simulink model "cx06_MA"  (Simulink 7.5)
settings: Solver=FixedStepDiscrete  StartTime=0.0  StopTime=10.0  RelTol=1e-3
undefined symbols (not defined in the file or in its folder): DiscIntNeverNeededParam, ECU555, int, motohawk_build_version, motohawk_trunc_name, motohawk_vardec_path
libraries: MotoHawk_lib x811, simulink x43, simulink_need_slupdate x1
(part 2 of 10)

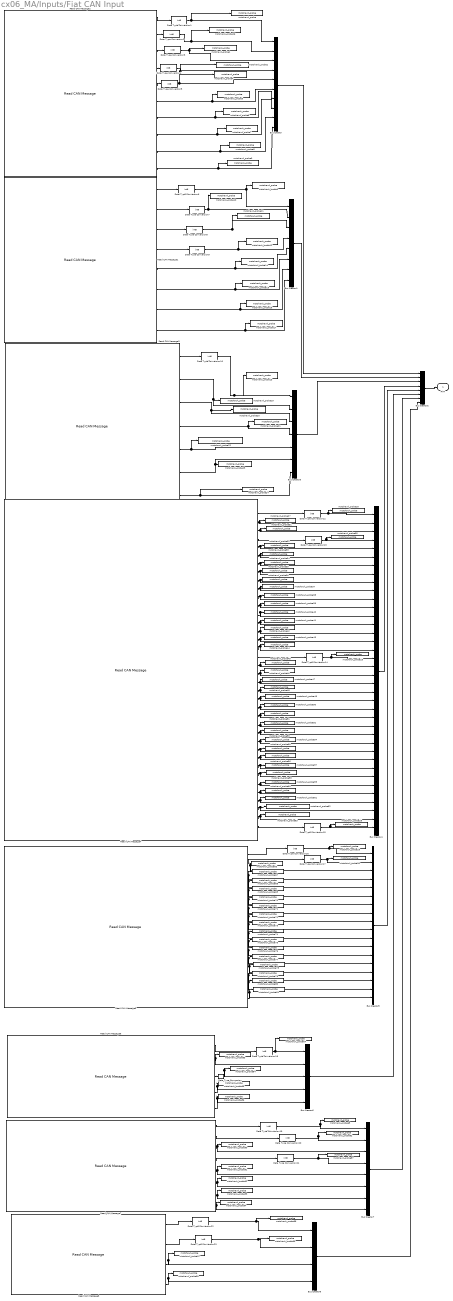
== system cx06_MA/Inputs/Fiat CAN Input ==
  Bus Creator : BusCreator  Inputs=10
  Bus Creator1 : BusCreator  Inputs=8
  Bus Creator2 : BusCreator  Inputs=8
  Bus Creator3 : BusCreator  Inputs=7
  Bus Creator4 : BusCreator  Inputs=38
  Bus Creator5 : BusCreator  Inputs=18
  Bus Creator6 : BusCreator  Inputs=5
  Bus Creator7 : BusCreator  Inputs=8
  Bus Creator8 : BusCreator
  Data Type Conversion : DataTypeConversion  OutDataTypeMode=uint8  OutDataType=sfix(16)  OutScaling=2^0  OutDataTypeStr=uint8
  Data Type Conversion{1..10,12..23} (22 alike) : DataTypeConversion  OutDataTypeMode=int8  OutDataType=sfix(16)  OutScaling=2^0  OutDataTypeStr=int8
  Read CAN Message1 : MotoHawk_lib/CAN Blocks/Read CAN Message  nam=['CAN_' num2str(1)]  bus=-2  msg=CANRx_FIAT_120  queue=2  slot=''  valid=off  stale=off  labelwires=on
  Read CAN Message2 : MotoHawk_lib/CAN Blocks/Read CAN Message  nam=['CAN_' num2str(1)]  bus=-2  msg=CANRx_FIAT_110  queue=2  slot=''  valid=off  stale=off  labelwires=on
  Read CAN Message3 : MotoHawk_lib/CAN Blocks/Read CAN Message  nam=['CAN_' num2str(1)]  bus=-2  msg=CANRx_FIAT_1A0  queue=2  slot=''  valid=off  stale=off  labelwires=on
  Read CAN Message4 : MotoHawk_lib/CAN Blocks/Read CAN Message  nam=['CAN_' num2str(1)]  bus=-2  msg=CANRx_FIAT_300  queue=2  slot=''  valid=off  stale=off  labelwires=on
  Read CAN Message5 : MotoHawk_lib/CAN Blocks/Read CAN Message  nam=['CAN_' num2str(1)]  bus=-2  msg=CANRx_FIAT_301  queue=2  slot=''  valid=off  stale=off  labelwires=on
  Read CAN Message6 : MotoHawk_lib/CAN Blocks/Read CAN Message  nam=['CAN_' num2str(1)]  bus=-2  msg=CANRx_FIAT_348  queue=2  slot=''  valid=off  stale=off  labelwires=on
  Read CAN Message7 : MotoHawk_lib/CAN Blocks/Read CAN Message  nam=['CAN_' num2str(1)]  bus=-2  msg=CANRx_FIAT_410  queue=2  slot=''  valid=off  stale=off  labelwires=on
  Read CAN Message8 : MotoHawk_lib/CAN Blocks/Read CAN Message  nam=['CAN_' num2str(1)]  bus=-2  msg=CANRx_FIAT_510  queue=2  slot=''  valid=off  stale=off  labelwires=on
  motohawk_probe{,1..3,10..13,18,25..26,28..30,64..65,82,87..89,95} (21 alike) : MotoHawk_lib/Calibration & Probing Blocks/motohawk_probe  nam='Probe'  show_more=on  name_source=Use Input Wire Name  read_level=1  view_as=Enumeration  enum_struct={'Valid', 'Invalid'}  vector_style=Wide Row  use_help_units=off  help=''  units=''  use_header_enum=off  row_header_enum={}  col_header_enum={}  use_precision=off  precision=''  gain=1  offset=0  exp=1  use_mototune_group=on  mototune_group=[motohawk_vardec_path(gcb), ' | Validities']
  motohawk_probe{5..8,14..17,19..20,24} (11 alike) : MotoHawk_lib/Calibration & Probing Blocks/motohawk_probe  nam='Probe'  show_more=off  name_source=Use Input Wire Name  read_level=1  view_as=Number  enum_struct={'Disabled', 'Enabled'}  vector_style=Wide Row  use_help_units=off  help=''  units=''  use_header_enum=off  row_header_enum={}  col_header_enum={}  use_precision=off  precision=''  gain=1  offset=0  exp=1  use_mototune_group=off  mototune_group=motohawk_vardec_path(gcb)
  motohawk_probe21 : MotoHawk_lib/Calibration & Probing Blocks/motohawk_probe  nam='Probe'  show_more=on  name_source=Use Input Wire Name  read_level=1  view_as=Number  enum_struct={'Status Unknown', 'Backup Mode Inactive', 'Backup Mode Active','Data Invalid'}  vector_style=Wide Row  use_help_units=off  help=''  units=''  use_header_enum=off  row_header_enum={}  col_header_enum={}  use_precision=off  precision=''  gain=1  offset=0  exp=1  use_mototune_group=off  mototune_group=motohawk_vardec_path(gcb)
  motohawk_probe22 : MotoHawk_lib/Calibration & Probing Blocks/motohawk_probe  nam='Probe'  show_more=on  name_source=Use Input Wire Name  read_level=1  view_as=Number  enum_struct={'Status Unknown', 'Normal Operation Without Failures','Reduced Power Mode Active','Power Management Mode Active','Safety Fuel Shut-Off Mode Active','Forced Idle Mode Active','Bowden Cable Mode Active','Engine Shut-Down Mode Active'}  vector_style=Wide Row  use_help_units=off  help=''  units=''  use_header_enum=off  row_header_enum={}  col_header_enum={}  use_precision=off  precision=''  gain=1  offset=0  exp=1  use_mototune_group=off  mototune_group=motohawk_vardec_path(gcb)
  motohawk_probe23 : MotoHawk_lib/Calibration & Probing Blocks/motohawk_probe  nam='Probe'  show_more=on  name_source=Use Input Wire Name  read_level=1  view_as=Number  enum_struct={'Status Unknown','Backup Mode Inactive','Backup Mode Active','Data Invalid'}  vector_style=Wide Row  use_help_units=off  help=''  units=''  use_header_enum=off  row_header_enum={}  col_header_enum={}  use_precision=off  precision=''  gain=1  offset=0  exp=1  use_mototune_group=off  mototune_group=motohawk_vardec_path(gcb)
  motohawk_probe{27,31..38,41..42,47..58,60..63,66..68,70..74,83,90..94,97..98} (43 alike) : MotoHawk_lib/Calibration & Probing Blocks/motohawk_probe  nam='Probe'  show_more=on  name_source=Use Input Wire Name  read_level=1  view_as=Number  enum_struct={'Valid','Invalid'}  vector_style=Wide Row  use_help_units=on  help=''  units=''  use_header_enum=off  row_header_enum={}  col_header_enum={}  use_precision=off  precision=''  gain=1  offset=0  exp=1  use_mototune_group=off  mototune_group=motohawk_vardec_path(gcb)
  motohawk_probe39 : MotoHawk_lib/Calibration & Probing Blocks/motohawk_probe  nam='Probe'  show_more=on  name_source=Use Input Wire Name  read_level=1  view_as=Number  enum_struct={'Not Running','Running and Idling','Running and Not Idling'}  vector_style=Wide Row  use_help_units=on  help=''  units=''  use_header_enum=off  row_header_enum={}  col_header_enum={}  use_precision=off  precision=''  gain=1  offset=0  exp=1  use_mototune_group=off  mototune_group=motohawk_vardec_path(gcb)
  motohawk_probe4 : MotoHawk_lib/Calibration & Probing Blocks/motohawk_probe  nam='Probe'  show_more=on  name_source=Use Input Wire Name  read_level=1  view_as=Enumeration  enum_struct={'Invalid','Valid'}  vector_style=Wide Row  use_help_units=off  help=''  units=''  use_header_enum=off  row_header_enum={}  col_header_enum={}  use_precision=off  precision=''  gain=1  offset=0  exp=1  use_mototune_group=on  mototune_group=[motohawk_vardec_path(gcb), ' | Validities']
  motohawk_probe40 : MotoHawk_lib/Calibration & Probing Blocks/motohawk_probe  nam='Probe'  show_more=on  name_source=Use Input Wire Name  read_level=1  view_as=Number  enum_struct={'Inactive','Active'}  vector_style=Wide Row  use_help_units=on  help=''  units=''  use_header_enum=off  row_header_enum={}  col_header_enum={}  use_precision=off  precision=''  gain=1  offset=0  exp=1  use_mototune_group=off  mototune_group=motohawk_vardec_path(gcb)
  motohawk_probe43 : MotoHawk_lib/Calibration & Probing Blocks/motohawk_probe  nam='Probe'  show_more=on  name_source=Use Input Wire Name  read_level=1  view_as=Number  enum_struct={'No Indication','Continuous Indication','Flashing Indication'}  vector_style=Wide Row  use_help_units=on  help=''  units=''  use_header_enum=off  row_header_enum={}  col_header_enum={}  use_precision=off  precision=''  gain=1  offset=0  exp=1  use_mototune_group=off  mototune_group=motohawk_vardec_path(gcb)
  motohawk_probe44 : MotoHawk_lib/Calibration & Probing Blocks/motohawk_probe  nam='Probe'  show_more=on  name_source=Use Input Wire Name  read_level=1  view_as=Number  enum_struct={'Cruise Not Active','Cruise Control In Command','Driver Overriding Cruise Command','Higher Priority Function Overriding'}  vector_style=Wide Row  use_help_units=on  help=''  units=''  use_header_enum=off  row_header_enum={}  col_header_enum={}  use_precision=off  precision=''  gain=1  offset=0  exp=1  use_mototune_group=off  mototune_group=motohawk_vardec_path(gcb)
  motohawk_probe45 : MotoHawk_lib/Calibration & Probing Blocks/motohawk_probe  nam='Probe'  show_more=on  name_source=Use Input Wire Name  read_level=1  view_as=Number  enum_struct={'Brake Not Applied','Brake Applied'}  vector_style=Wide Row  use_help_units=on  help=''  units=''  use_header_enum=off  row_header_enum={}  col_header_enum={}  use_precision=off  precision=''  gain=1  offset=0  exp=1  use_mototune_group=off  mototune_group=motohawk_vardec_path(gcb)
  motohawk_probe46 : MotoHawk_lib/Calibration & Probing Blocks/motohawk_probe  nam='Probe'  show_more=on  name_source=Use Input Wire Name  read_level=1  view_as=Number  enum_struct={'Brake Not Applied','Brake Applied'}  vector_style=Wide Row  use_help_units=on  help=''  units=''  use_header_enum=off  row_header_enum={}  col_header_enum={}  use_precision=off  precision=''  gain=1  offset=0  exp=1  use_mototune_group=off  mototune_group=motohawk_vardec_path(gcb)
  motohawk_probe59 : MotoHawk_lib/Calibration & Probing Blocks/motohawk_probe  nam='Probe'  show_more=on  name_source=Use Input Wire Name  read_level=1  view_as=Number  enum_struct={'Limited Slip Control Permitted','Limited Slip Control Inhibited'}  vector_style=Wide Row  use_help_units=on  help=''  units=''  use_header_enum=off  row_header_enum={}  col_header_enum={}  use_precision=off  precision=''  gain=1  offset=0  exp=1  use_mototune_group=off  mototune_group=motohawk_vardec_path(gcb)
  motohawk_probe69 : MotoHawk_lib/Calibration & Probing Blocks/motohawk_probe  nam='Probe'  show_more=on  name_source=Use Input Wire Name  read_level=1  view_as=Number  enum_struct={'None','Shift Up','Shift Down','Neutral'}  vector_style=Wide Row  use_help_units=on  help=''  units=''  use_header_enum=off  row_header_enum={}  col_header_enum={}  use_precision=off  precision=''  gain=1  offset=0  exp=1  use_mototune_group=off  mototune_group=motohawk_vardec_path(gcb)
  motohawk_probe75 : MotoHawk_lib/Calibration & Probing Blocks/motohawk_probe  nam='Probe'  show_more=on  name_source=Use Input Wire Name  read_level=1  view_as=Number  enum_struct={'No Request','Inhibit Gear Shift'}  vector_style=Wide Row  use_help_units=on  help=''  units=''  use_header_enum=off  row_header_enum={}  col_header_enum={}  use_precision=off  precision=''  gain=1  offset=0  exp=1  use_mototune_group=off  mototune_group=motohawk_vardec_path(gcb)
  motohawk_probe76 : MotoHawk_lib/Calibration & Probing Blocks/motohawk_probe  nam='Probe'  show_more=on  name_source=Use Input Wire Name  read_level=1  view_as=Number  enum_struct={'No Request','Request Jerk Shift Pattern'}  vector_style=Wide Row  use_help_units=on  help=''  units=''  use_header_enum=off  row_header_enum={}  col_header_enum={}  use_precision=off  precision=''  gain=1  offset=0  exp=1  use_mototune_group=off  mototune_group=motohawk_vardec_path(gcb)
  motohawk_probe77 : MotoHawk_lib/Calibration & Probing Blocks/motohawk_probe  nam='Probe'  show_more=on  name_source=Use Input Wire Name  read_level=1  view_as=Number  enum_struct={'No Request','Inhibit Neutral Control'}  vector_style=Wide Row  use_help_units=on  help=''  units=''  use_header_enum=off  row_header_enum={}  col_header_enum={}  use_precision=off  precision=''  gain=1  offset=0  exp=1  use_mototune_group=off  mototune_group=motohawk_vardec_path(gcb)
  motohawk_probe78 : MotoHawk_lib/Calibration & Probing Blocks/motohawk_probe  nam='Probe'  show_more=on  name_source=Use Input Wire Name  read_level=1  view_as=Number  enum_struct={'No Request','Request REP Shift Pattern'}  vector_style=Wide Row  use_help_units=on  help=''  units=''  use_header_enum=off  row_header_enum={}  col_header_enum={}  use_precision=off  precision=''  gain=1  offset=0  exp=1  use_mototune_group=off  mototune_group=motohawk_vardec_path(gcb)
  motohawk_probe79 : MotoHawk_lib/Calibration & Probing Blocks/motohawk_probe  nam='Probe'  show_more=on  name_source=Use Input Wire Name  read_level=1  view_as=Number  enum_struct={'Map A','Map B','Map C','ECM Selected Progression'}  vector_style=Wide Row  use_help_units=on  help=''  units=''  use_header_enum=off  row_header_enum={}  col_header_enum={}  use_precision=off  precision=''  gain=1  offset=0  exp=1  use_mototune_group=off  mototune_group=motohawk_vardec_path(gcb)
  motohawk_probe80 : MotoHawk_lib/Calibration & Probing Blocks/motohawk_probe  nam='Probe'  show_more=on  name_source=Use Input Wire Name  read_level=1  view_as=Number  enum_struct={'Map A','Map B','Map C','ECM Selected Progression'}  vector_style=Wide Row  use_help_units=on  help=''  units=''  use_header_enum=off  row_header_enum={}  col_header_enum={}  use_precision=off  precision=''  gain=1  offset=0  exp=1  use_mototune_group=off  mototune_group=motohawk_vardec_path(gcb)
  motohawk_probe81 : MotoHawk_lib/Calibration & Probing Blocks/motohawk_probe  nam='Probe'  show_more=on  name_source=Use Input Wire Name  read_level=1  view_as=Number  enum_struct={'Map A','Map B','Map C','ECM Selected Progression'}  vector_style=Wide Row  use_help_units=on  help=''  units=''  use_header_enum=off  row_header_enum={}  col_header_enum={}  use_precision=off  precision=''  gain=1  offset=0  exp=1  use_mototune_group=off  mototune_group=motohawk_vardec_path(gcb)
  motohawk_probe84 : MotoHawk_lib/Calibration & Probing Blocks/motohawk_probe  nam='Probe'  show_more=on  name_source=Use Input Wire Name  read_level=1  view_as=Enumeration  enum_struct={'No Action','Engage','Minimum Stroke','Security Shutdown'}  vector_style=Wide Row  use_help_units=on  help=''  units=''  use_header_enum=off  row_header_enum={}  col_header_enum={}  use_precision=off  precision=''  gain=1  offset=0  exp=1  use_mototune_group=off  mototune_group=motohawk_vardec_path(gcb)
  motohawk_probe85 : MotoHawk_lib/Calibration & Probing Blocks/motohawk_probe  nam='Probe'  show_more=on  name_source=Use Input Wire Name  read_level=1  view_as=Number  enum_struct={'No Action','Engage','Minimum Stroke','Security Shutdown'}  vector_style=Wide Row  use_help_units=on  help=''  units=''  use_header_enum=off  row_header_enum={}  col_header_enum={}  use_precision=off  precision=''  gain=1  offset=0  exp=1  use_mototune_group=off  mototune_group=motohawk_vardec_path(gcb)
  motohawk_probe86 : MotoHawk_lib/Calibration & Probing Blocks/motohawk_probe  nam='Probe'  show_more=on  name_source=Use Input Wire Name  read_level=1  view_as=Number  enum_struct={'No Action','Engage','Minimum Stroke','Security Shutdown'}  vector_style=Wide Row  use_help_units=on  help=''  units=''  use_header_enum=off  row_header_enum={}  col_header_enum={}  use_precision=off  precision=''  gain=1  offset=0  exp=1  use_mototune_group=off  mototune_group=motohawk_vardec_path(gcb)
  motohawk_probe9 : MotoHawk_lib/Calibration & Probing Blocks/motohawk_probe  nam='Probe'  show_more=on  name_source=Use Input Wire Name  read_level=1  view_as=Number  enum_struct={'Disabled', 'Enabled'}  vector_style=Wide Row  use_help_units=off  help=''  units=''  use_header_enum=off  row_header_enum={}  col_header_enum={}  use_precision=off  precision=''  gain=1  offset=0  exp=1  use_mototune_group=off  mototune_group=motohawk_vardec_path(gcb)
  FIAT : Outport  OutDataType=sfix(16)  OutScaling=2^0
  wires:
  Read CAN Message2/1 -> Data Type Conversion1/1  "Eng_Spd_V"
  Read CAN Message2/2 -> Data Type Conversion2/1  "Acel_Effect_Pos_V"
  Read CAN Message2/3 -> Data Type Conversion3/1  "Acel_Grad_V"
  Read CAN Message2/4 -> Data Type Conversion4/1  "Throt_Pos_V"
  Bus Creator/1 -> Bus Creator2/1  "Engine Speed and Pedal Pos"
  Bus Creator2/1 -> FIAT/1
  Read CAN Message2/5 -> Data Type Conversion5/1  "Acel_Actual_Pos_V"
  Read CAN Message2/7 -> Bus Creator/7, motohawk_probe6/1  "Acel_Effect_Pos"
  Read CAN Message2/8 -> Bus Creator/8, motohawk_probe7/1  "Acel_Grad"
  Read CAN Message2/9 -> Bus Creator/9, motohawk_probe8/1  "Throt_Pos"
  Read CAN Message2/10 -> Bus Creator/10, motohawk_probe9/1  "Acel_Actual_Pos"
  Read CAN Message1/1 -> Data Type Conversion6/1  "Eng_Torq_Actual_V"
  Read CAN Message1/2 -> Data Type Conversion7/1  "Eng_Torq_Driver_Reqest_V"
  Read CAN Message1/3 -> Data Type Conversion8/1  "Eng_Max_Drag_Torq_V"
  Read CAN Message1/4 -> Data Type Conversion9/1  "Eng_Torq_Max_V"
  Read CAN Message1/5 -> Bus Creator1/5, motohawk_probe14/1  "Eng_Torq_Actual"
  Read CAN Message1/6 -> Bus Creator1/6, motohawk_probe15/1  "Eng_Torq_Request"
  Read CAN Message1/7 -> Bus Creator1/7, motohawk_probe16/1  "Eng_Max_Drag_Torq"
  Read CAN Message1/8 -> Bus Creator1/8, motohawk_probe17/1  "Eng_Torq_Max"
  Bus Creator1/1 -> Bus Creator2/2  "Engine Torque"
  Read CAN Message2/6 -> Bus Creator/6, motohawk_probe5/1  "Eng_Spd"
  Read CAN Message3/1 -> Data Type Conversion10/1  "Eng_Idle_Spd_V"
  Read CAN Message3/2 -> Bus Creator3/2, motohawk_probe19/1  "Eng_Idle_Spd"
  Read CAN Message3/3 -> Bus Creator3/3, motohawk_probe20/1  "Base_Target_Eng_Idle_Spd"
  Read CAN Message3/4 -> Bus Creator3/4, motohawk_probe21/1  "Eng_Airflow_Backup_Mode"
  Read CAN Message3/5 -> Bus Creator3/5, motohawk_probe22/1  "Eng_Throt_Control_Operat"
  Read CAN Message3/6 -> Bus Creator3/6, motohawk_probe23/1  "Eng_Crankshaft_Backup_Mode"
  Read CAN Message3/7 -> Bus Creator3/7, motohawk_probe24/1  "Eng_Allowed_Clutch_Adapt"
  Bus Creator3/1 -> Bus Creator2/3  "Engine Idle Speed Info"
  Read CAN Message4/1 -> Data Type Conversion12/1  "Brake_Ped_Switch_Active_V"
  Read CAN Message4/2 -> Bus Creator4/2, motohawk_probe27/1  "Part_Filter_Clean_Alg_Active"
  Read CAN Message4/3 -> Bus Creator4/3, motohawk_probe31/1  "Fuel_Inj_Roll_Cnt_Reset_Occured"
  Read CAN Message4/5 -> Bus Creator4/5, motohawk_probe32/1  "Eng_Limp_Home_Mode"
  Read CAN Message4/6 -> Bus Creator4/6, motohawk_probe33/1  "Eng_Torq_Reduction_Failed"
  Read CAN Message4/7 -> Bus Creator4/7, motohawk_probe34/1  "Eng_Fail_Code_Retrieval_Required"
  Read CAN Message4/8 -> Bus Creator4/8, motohawk_probe35/1  "Generator_Failed"
  Read CAN Message4/9 -> Bus Creator4/9, motohawk_probe36/1  "Brake_Ped_Switch"
  Read CAN Message4/10 -> Bus Creator4/10, motohawk_probe37/1  "Cruise_Control_Clutch_Switch"
  Read CAN Message4/11 -> Bus Creator4/11, motohawk_probe38/1  "Cruise_Control_Active"
  Read CAN Message4/12 -> Bus Creator4/12, motohawk_probe39/1  "Eng_Running_Stat"
  Read CAN Message4/13 -> Bus Creator4/13, motohawk_probe40/1  "Warm_Up_Shift_Pattern_Req"
  Read CAN Message4/14 -> Bus Creator4/14, motohawk_probe41/1  "Rough_Road"
  Read CAN Message4/15 -> Bus Creator4/15, motohawk_probe42/1  "Eng_Warm_Up_Cycle_Achieved"
  Read CAN Message4/16 -> Bus Creator4/16, motohawk_probe43/1  "Service_Eng_Non_Emission"
  Read CAN Message4/17 -> Bus Creator4/17, motohawk_probe44/1  "Cruise_Control_Throt_Cmd_Stat"
  Read CAN Message4/19 -> Bus Creator4/19, motohawk_probe45/1  "PwrTrn_Brk_Ped_Sec_In"
  Read CAN Message4/20 -> Bus Creator4/20, motohawk_probe46/1  "PrwTrn_Brk_Ped_In"
  Read CAN Message4/21 -> Bus Creator4/21, motohawk_probe47/1  "Eng_Oil_Lvl_Low"
  Read CAN Message4/22 -> Bus Creator4/22, motohawk_probe48/1  "Eng_Oil_Pres_Low"
  Read CAN Message4/23 -> Bus Creator4/23, motohawk_probe49/1  "Accel_Kick_Down"
  Read CAN Message4/24 -> motohawk_probe50/1, Bus Creator4/24  "Glow_Plug"
  Read CAN Message4/25 -> Bus Creator4/25, motohawk_probe51/1  "PrwTrn_Crank"
  Read CAN Message4/26 -> Bus Creator4/26, motohawk_probe52/1  "Eng_Trans_Emission_DTC_Stored"
  Read CAN Message4/27 -> Bus Creator4/27, motohawk_probe53/1  "Eng_Torq_Tract_Control_Req_Failed"
  Read CAN Message4/28 -> Bus Creator4/28, motohawk_probe54/1  "Eng_Torq_Trans_Req_Failed"
  Read CAN Message4/29 -> Bus Creator4/29, motohawk_probe55/1  "Fuel_Inj_Roll_Cnt"
  Read CAN Message4/30 -> Bus Creator4/30, motohawk_probe56/1  "Fuel_Lvl_Sensor_Unprocessed"
  Read CAN Message4/31 -> Bus Creator4/31, motohawk_probe57/1  "Eng_Emissions_Malfunction"
  Read CAN Message4/32 -> Bus Creator4/32, motohawk_probe58/1  "Cruise_Control_Enabled"
  Read CAN Message4/33 -> Bus Creator4/33, motohawk_probe59/1  "Eng_Coast_Limit_Slip"
  Read CAN Message4/34 -> Bus Creator4/34, motohawk_probe60/1  "Eng_Oil_Change_Now"
  Read CAN Message4/35 -> Bus Creator4/35, motohawk_probe61/1  "Eng_Oil_Change_Soon"
  Read CAN Message4/36 -> Bus Creator4/36, motohawk_probe62/1  "Eng_Coast_Fuel_Cut_Off_Active"
  Read CAN Message4/37 -> Bus Creator4/37, motohawk_probe63/1  "Eng_Torq_Cruise_Control_Req_Failed"
  Read CAN Message4/38 -> Data Type Conversion15/1  "PwrTrn_Brk_Ped_In_V"
  Read CAN Message4/4 -> Data Type Conversion13/1  "Fuel_Lvl_Sensor_Unprocessed_Value_V"
  Read CAN Message5/2 -> Data Type Conversion17/1  "Baro_Pres_Abs_V"
  Read CAN Message5/3 -> motohawk_probe66/1, Bus Creator5/3  "PwrTrn_Hi_Elect_Load_Req"
  Read CAN Message5/4 -> motohawk_probe67/1, Bus Creator5/4  "Aply_Brk_Pedal_Ind"
  Read CAN Message5/5 -> motohawk_probe68/1, Bus Creator5/5  "Check_Fuel_Cap"
  Read CAN Message5/6 -> motohawk_probe69/1, Bus Creator5/6  "Eng_Recommend_Shft"
  Read CAN Message5/7 -> motohawk_probe70/1, Bus Creator5/7  "Eng_H20_In_Fuel"
  Read CAN Message5/8 -> motohawk_probe71/1, Bus Creator5/8  "Eng_Boost_Pres"
  Read CAN Message5/9 -> motohawk_probe72/1, Bus Creator5/9  "Eng_Oil_Remaining_Life"
  Read CAN Message5/10 -> motohawk_probe73/1, Bus Creator5/10  "Eng_Prod_Option_Ident"
  Read CAN Message5/11 -> motohawk_probe74/1, Bus Creator5/11  "Eng_Fan_Spd"
  Read CAN Message5/12 -> motohawk_probe75/1, Bus Creator5/12  "Eng_Gear_Shift_Inh_Req"
  Read CAN Message5/13 -> motohawk_probe76/1, Bus Creator5/13  "Eng_Jerk_Shift_Pattern_Req"
  Read CAN Message5/14 -> motohawk_probe77/1, Bus Creator5/14  "Eng_Ntral_Control_Inh_Req"
  Read CAN Message5/15 -> motohawk_probe78/1, Bus Creator5/15  "Reduce_Prf_Shft_Ptrn_Req"
  Read CAN Message5/16 -> motohawk_probe79/1, Bus Creator5/16  "Throt_Progression"
  Read CAN Message5/17 -> motohawk_probe80/1, Bus Creator5/17  "PwrTrn_Part_Filter Warning"
  Read CAN Message5/18 -> motohawk_probe81/1, Bus Creator5/18  "Baro_Pres_Abs"
  Read CAN Message6/1 -> Data Type Conversion18/1  "AC_Ref_Hi_Side_Pres_V"
  Read CAN Message6/2 -> motohawk_probe83/1, Bus Creator6/2  "AC_Comp_Clutch_Engaged"
  Read CAN Message6/3 -> Data Type Conversion/1  "AC_Comp_Stroke_Req"
  Read CAN Message6/4 -> motohawk_probe85/1, Bus Creator6/4  "AC_Off_Ind"
  Read CAN Message6/5 -> motohawk_probe86/1, Bus Creator6/5  "AC_Ref_Hi_Side_Pres"
  Read CAN Message7/1 -> Data Type Conversion19/1  "Veh_Spd_V"
  Read CAN Message7/2 -> Data Type Conversion20/1  "Dist_Roll_Cnt_Lft_V"
  Read CAN Message7/4 -> Data Type Conversion21/1  "Dist_Roll_Cnt_Rht_V"
  Read CAN Message7/3 -> motohawk_probe90/1, Bus Creator7/3  "Dist_Roll_Cnt_Lft_Reset"
  Read CAN Message7/5 -> motohawk_probe91/1, Bus Creator7/5  "Dist_Roll_Cnt_Rht_Reset"
  Read CAN Message7/6 -> motohawk_probe92/1, Bus Creator7/6  "Veh_Spd"
  Read CAN Message7/7 -> motohawk_probe93/1, Bus Creator7/7  "Dist_Roll_Cnt_Lft"
  Read CAN Message7/8 -> motohawk_probe94/1, Bus Creator7/8  "Dist_Roll_Cnt_Rht"
  Read CAN Message8/3 -> motohawk_probe97/1, Bus Creator8/3  "Eng_Coolant_Temp"
  Read CAN Message8/4 -> motohawk_probe98/1, Bus Creator8/4  "Eng_Intake_Air_Temp"
  Bus Creator4/1 -> Bus Creator2/4  "Engine  General Status"
  Bus Creator5/1 -> Bus Creator2/5  "Engine General Status 2"
  Bus Creator6/1 -> Bus Creator2/6  "Engine AC Status"
  Bus Creator7/1 -> Bus Creator2/7  "Vehicle Speed and Odometer"
  Bus Creator8/1 -> Bus Creator2/8  "Engine Temp"
  Data Type Conversion/1 -> motohawk_probe84/1, Bus Creator6/3  "AC_Comp_Stroke_Req"
  Data Type Conversion1/1 -> Bus Creator/1, motohawk_probe/1  "Eng_Spd_V"
  Data Type Conversion2/1 -> Bus Creator/2, motohawk_probe26/1  "Acel_Effect_Pos_V"
  Data Type Conversion3/1 -> Bus Creator/3, motohawk_probe1/1  "Acel_Grad_V"
  Data Type Conversion4/1 -> Bus Creator/4, motohawk_probe2/1  "Throt_Pos_V"
  Data Type Conversion5/1 -> Bus Creator/5, motohawk_probe4/1  "Acel_Actual_Pos_V"
  Data Type Conversion6/1 -> Bus Creator1/1, motohawk_probe3/1  "Eng_Torq_Actual_V"
  Data Type Conversion7/1 -> Bus Creator1/2, motohawk_probe10/1  "Eng_Torq_Driver_Reqest_V"
  Data Type Conversion8/1 -> Bus Creator1/3, motohawk_probe11/1  "Eng_Max_Drag_Torq_V"
  Data Type Conversion9/1 -> Bus Creator1/4, motohawk_probe12/1  "Eng_Torq_Max_V"
  Data Type Conversion10/1 -> Bus Creator3/1, motohawk_probe13/1  "Eng_Idle_Spd_V"
  Data Type Conversion12/1 -> Bus Creator4/1, motohawk_probe18/1  "Brake_Ped_Switch_Active_V"
  Data Type Conversion13/1 -> Bus Creator4/4, motohawk_probe95/1  "Fuel_Lvl_Sensor_Unprocessed_Value_V"
  Read CAN Message4/18 -> Data Type Conversion14/1  "PwrTrn_Brk_Ped_Sec_In_V"
  Data Type Conversion14/1 -> Bus Creator4/18, motohawk_probe25/1  "PwrTrn_Brk_Ped_Sec_In_V"
  Data Type Conversion15/1 -> Bus Creator4/38, motohawk_probe28/1  "PwrTrn_Brk_Ped_In_V"
  Read CAN Message5/1 -> Data Type Conversion16/1  "Eng_Boost_Pres_V"
  Data Type Conversion16/1 -> Bus Creator5/1, motohawk_probe29/1  "Eng_Boost_Pres_V"
  Data Type Conversion17/1 -> Bus Creator5/2, motohawk_probe30/1  "Baro_Pres_Abs_V"
  Data Type Conversion18/1 -> Bus Creator6/1, motohawk_probe64/1  "AC_Ref_Hi_Side_Pres_V"
  Data Type Conversion19/1 -> Bus Creator7/1, motohawk_probe65/1  "Veh_Spd_V"
  Data Type Conversion20/1 -> Bus Creator7/2, motohawk_probe82/1  "Dist_Roll_Cnt_Lft_V"
  Data Type Conversion21/1 -> Bus Creator7/4, motohawk_probe87/1  "Dist_Roll_Cnt_Rht_V"
  Read CAN Message8/1 -> Data Type Conversion22/1  "Eng_Coolant_Temp_V"
  Data Type Conversion22/1 -> Bus Creator8/1, motohawk_probe88/1  "Eng_Coolant_Temp_V"
  Read CAN Message8/2 -> Data Type Conversion23/1  "Eng_Intake_Air_Temp_V"
  Data Type Conversion23/1 -> Bus Creator8/2, motohawk_probe89/1  "Eng_Intake_Air_Temp_V"

== system cx06_MA/Inputs/GMLAN Inputs ==
  Bus Creator : BusCreator  Inputs=10
  Compare To Constant1 : simulink/Logic and Bit Operations/Compare To Constant  SystemSampleTime=-1  relop=>  const=10  LogicOutDataTypeMode=boolean  ZeroCross=off
  Compare To Constant2 : simulink/Logic and Bit Operations/Compare To Constant  SystemSampleTime=-1  relop=>  const=20  LogicOutDataTypeMode=boolean  ZeroCross=off
  Read CAN Message : MotoHawk_lib/CAN Blocks/Read CAN Message  nam=['CAN_' num2str(2)]  bus=-2  msg=CANRx_GMLAN_280  queue=1  slot=''  valid=off  stale=on  labelwires=on
  Read CAN Message1 : MotoHawk_lib/CAN Blocks/Read CAN Message  nam=['CAN_' num2str(2)]  bus=-2  msg=CANRx_GMLAN_380  queue=1  slot=''  valid=off  stale=on  labelwires=on
  Valid_Chk : Subsystem
  Valid_Chk1 : Subsystem
  Valid_Chk2 : Subsystem
  Valid_Chk3 : Subsystem
  motohawk_fault_def1 : MotoHawk_lib/Fault Management Blocks/motohawk_fault_def  nam='GMLAN380'  mode=Enabled - Persistent  id=[]  x=10  y=11  input_suspected=on  indeterminate=off  increment_xy=on  downsample_count=1  ovr_cals=on  ovr_actions=on  show_actions=on  action1_name=''  action1_cond=(None)  action2_name=''  action2_cond=(None)  action3_name=''  action3_cond=(None)  action4_name=''  action4_cond=(None)
  motohawk_fault_def2 : MotoHawk_lib/Fault Management Blocks/motohawk_fault_def  nam='GMLAN280'  mode=Enabled - Persistent  id=[]  x=10  y=11  input_suspected=on  indeterminate=off  increment_xy=on  downsample_count=1  ovr_cals=on  ovr_actions=on  show_actions=on  action1_name=''  action1_cond=(None)  action2_name=''  action2_cond=(None)  action3_name=''  action3_cond=(None)  action4_name=''  action4_cond=(None)
  motohawk_probe{,1..12} (13 alike) : MotoHawk_lib/Calibration & Probing Blocks/motohawk_probe  nam='Probe'  show_more=on  name_source=Use Input Wire Name  read_level=1  view_as=Number  enum_struct={'Disabled', 'Enabled'}  vector_style=Wide Row  use_help_units=off  help=''  units=''  use_header_enum=off  row_header_enum={}  col_header_enum={}  use_precision=off  precision=''  gain=1  offset=0  exp=1  use_mototune_group=off  mototune_group=motohawk_vardec_path(gcb)
  GMLAN : Outport  OutDataType=sfix(16)  OutScaling=2^0
  wires:
  Valid_Chk/1(Out1) -> Bus Creator/2  "FL_Whl_Spd"
  Valid_Chk1/1(Out1) -> Bus Creator/3  "FR_Whl_Spd"
  Valid_Chk2/1(Out1) -> Bus Creator/4  "RL_Whl_Spd"
  Valid_Chk3/1(Out1) -> Bus Creator/5  "RR_Whl_Spd"
  Compare To Constant2/1 -> motohawk_fault_def2/1  "AgeCount"
  Read CAN Message/1 -> Compare To Constant2/1, Bus Creator/1  "AgeCount"
  Read CAN Message/2 -> motohawk_probe/1, Valid_Chk/1(In)  "FL_Wheel_Vel"
  Read CAN Message/3 -> motohawk_probe1/1, Valid_Chk/2(Valid)  "FL_Wheel_Valid"
  Read CAN Message/4 -> motohawk_probe2/1, Valid_Chk1/1(In)  "FR_Wheel_Vel"
  Read CAN Message/5 -> motohawk_probe3/1, Valid_Chk1/2(Valid)  "FR_Wheel_Valid"
  Read CAN Message/6 -> motohawk_probe4/1, Valid_Chk2/1(In)  "RL_Wheel_Vel"
  Read CAN Message/7 -> motohawk_probe5/1, Valid_Chk2/2(Valid)  "RL_Wheel_Valid"
  Read CAN Message/8 -> motohawk_probe6/1, Valid_Chk3/1(In)  "RR_Wheel_Vel"
  Read CAN Message/9 -> motohawk_probe7/1, Valid_Chk3/2(Valid)  "RR_Wheel_Valid"
  Compare To Constant1/1 -> motohawk_fault_def1/1  "AgeCount"
  Read CAN Message1/1 -> Compare To Constant1/1  "AgeCount"
  Read CAN Message1/2 -> motohawk_probe8/1, Bus Creator/6  "AC_Clutch_Req"
  Read CAN Message1/3 -> motohawk_probe9/1, Bus Creator/7  "System_Power_Mode"
  Read CAN Message1/4 -> motohawk_probe10/1, Bus Creator/8  "RunCrank_Status"
  Read CAN Message1/5 -> motohawk_probe11/1, Bus Creator/9  "Acc_Status"
  Bus Creator/1 -> GMLAN/1  "GMLAN"
  Read CAN Message1/6 -> Bus Creator/10, motohawk_probe12/1  "Park_Brake"

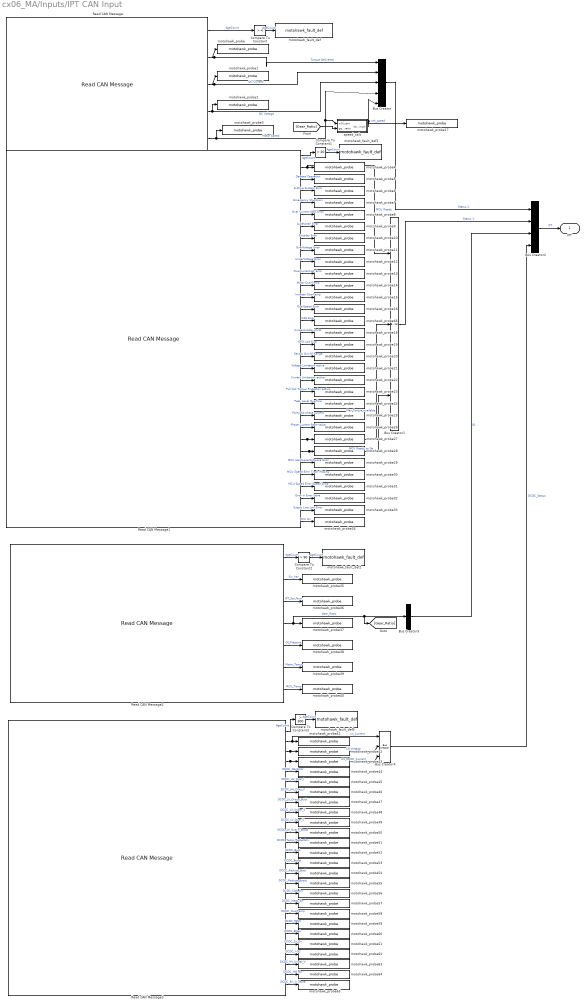
== system cx06_MA/Inputs/IPT CAN Input ==
  Bus Creator : BusCreator  Inputs=5
  Bus Creator1 : BusCreator  Inputs=3
  Bus Creator2 : BusCreator
  Bus Creator3 : BusCreator  Inputs=1
  Bus Creator4 : BusCreator  Inputs=3
  Compare To Constant : simulink/Logic and Bit Operations/Compare To Constant  SystemSampleTime=-1  relop=>  const=4  LogicOutDataTypeMode=boolean  ZeroCross=off
  Compare To Constant1 : simulink/Logic and Bit Operations/Compare To Constant  SystemSampleTime=-1  relop=>  const=20  LogicOutDataTypeMode=boolean  ZeroCross=off
  Compare To Constant2 : simulink/Logic and Bit Operations/Compare To Constant  SystemSampleTime=-1  relop=>  const=90  LogicOutDataTypeMode=boolean  ZeroCross=off
  Compare To Constant3 : simulink/Logic and Bit Operations/Compare To Constant  SystemSampleTime=-1  relop=>  const=300  LogicOutDataTypeMode=boolean  ZeroCross=off
  Read CAN Message : MotoHawk_lib/CAN Blocks/Read CAN Message  nam=['CAN_' num2str(1)]  bus=-2  msg=CANRx_IPT_258  queue=2  slot=''  valid=off  stale=on  labelwires=on
  Read CAN Message1 : MotoHawk_lib/CAN Blocks/Read CAN Message  nam=['CAN_' num2str(1)]  bus=-2  msg=CANRx_IPT_278  queue=2  slot=''  valid=off  stale=on  labelwires=on
  Read CAN Message2 : MotoHawk_lib/CAN Blocks/Read CAN Message  nam=['CAN_' num2str(1)]  bus=-2  msg=CANRx_IPT_638  queue=1  slot=''  valid=off  stale=on  labelwires=on
  Read CAN Message3 : MotoHawk_lib/CAN Blocks/Read CAN Message  nam=['CAN_' num2str(1)]  bus=-2  msg=CANRx_IPT_620  queue=1  slot=''  valid=off  stale=on  labelwires=on
  motohawk_fault_def : MotoHawk_lib/Fault Management Blocks/motohawk_fault_def  nam='IPT258'  mode=Enabled - Persistent  id=[]  x=10  y=11  input_suspected=on  indeterminate=off  increment_xy=on  downsample_count=1  ovr_cals=on  ovr_actions=on  show_actions=on  action1_name=''  action1_cond=Active  action2_name='inhibitEV'  action2_cond=Active  action3_name=''  action3_cond=(None)  action4_name=''  action4_cond=(None)
  motohawk_fault_def1 : MotoHawk_lib/Fault Management Blocks/motohawk_fault_def  nam='IPT278'  mode=Enabled - Persistent  id=[]  x=10  y=11  input_suspected=on  indeterminate=off  increment_xy=on  downsample_count=1  ovr_cals=on  ovr_actions=on  show_actions=on  action1_name=''  action1_cond=Active  action2_name='inhibitEV'  action2_cond=Active  action3_name=''  action3_cond=(None)  action4_name=''  action4_cond=(None)
  motohawk_fault_def2 : MotoHawk_lib/Fault Management Blocks/motohawk_fault_def  nam='IPT638'  mode=Enabled - Persistent  id=[]  x=10  y=11  input_suspected=on  indeterminate=off  increment_xy=on  downsample_count=1  ovr_cals=on  ovr_actions=on  show_actions=on  action1_name='inhibitEV'  action1_cond=Active  action2_name=''  action2_cond=(None)  action3_name=''  action3_cond=(None)  action4_name=''  action4_cond=(None)
  motohawk_fault_def3 : MotoHawk_lib/Fault Management Blocks/motohawk_fault_def  nam='IPT620'  mode=Enabled - Persistent  id=[]  x=29  y=30  input_suspected=on  indeterminate=off  increment_xy=on  downsample_count=1  ovr_cals=on  ovr_actions=on  show_actions=on  action1_name=''  action1_cond=Active  action2_name=''  action2_cond=(None)  action3_name=''  action3_cond=(None)  action4_name=''  action4_cond=(None)
  motohawk_probe : MotoHawk_lib/Calibration & Probing Blocks/motohawk_probe  nam='Probe'  show_more=on  name_source=Use Input Wire Name  read_level=1  view_as=Number  enum_struct={'Disabled', 'Enabled'}  vector_style=Wide Row  use_help_units=off  help=''  units=''  use_header_enum=off  row_header_enum={}  col_header_enum={}  use_precision=off  precision=''  gain=1  offset=0  exp=1  use_mototune_group=off  mototune_group=motohawk_vardec_path(gcb)
  motohawk_probe1 : MotoHawk_lib/Calibration & Probing Blocks/motohawk_probe  nam='Probe'  show_more=on  name_source=Use Input Wire Name  read_level=1  view_as=Number  enum_struct={'Disabled', 'Enabled'}  vector_style=Wide Row  use_help_units=off  help=''  units=''  use_header_enum=off  row_header_enum={}  col_header_enum={}  use_precision=off  precision=''  gain=1  offset=0  exp=1  use_mototune_group=off  mototune_group=motohawk_vardec_path(gcb)
  motohawk_probe{3..16,18..66} (63 alike) : MotoHawk_lib/Calibration & Probing Blocks/motohawk_probe  nam='Probe'  show_more=off  name_source=Use Input Wire Name  read_level=1  view_as=Number  enum_struct={'Disabled', 'Enabled'}  vector_style=Wide Row  use_help_units=off  help=''  units=''  use_header_enum=off  row_header_enum={}  col_header_enum={}  use_precision=off  precision=''  gain=1  offset=0  exp=1  use_mototune_group=off  mototune_group=motohawk_vardec_path(gcb)
  motohawk_probe17 : MotoHawk_lib/Calibration & Probing Blocks/motohawk_probe  nam='vehicle_speed'  show_more=on  name_source=Use Parameter  read_level=1  view_as=Number  enum_struct={'Disabled', 'Enabled'}  vector_style=Wide Row  use_help_units=off  help=''  units=''  use_header_enum=off  row_header_enum={}  col_header_enum={}  use_precision=off  precision=''  gain=1  offset=0  exp=1  use_mototune_group=off  mototune_group=motohawk_vardec_path(gcb)
  motohawk_probe2 : MotoHawk_lib/Calibration & Probing Blocks/motohawk_probe  nam='Probe'  show_more=on  name_source=Use Input Wire Name  read_level=1  view_as=Number  enum_struct={'Disabled', 'Enabled'}  vector_style=Wide Row  use_help_units=off  help=''  units=''  use_header_enum=off  row_header_enum={}  col_header_enum={}  use_precision=off  precision=''  gain=1  offset=0  exp=1  use_mototune_group=off  mototune_group=motohawk_vardec_path(gcb)
  speed_calc : Subsystem
  IPT : Outport  OutDataType=sfix(16)  OutScaling=2^0
  wires:
  Bus Creator/1 -> Bus Creator2/1  "Status 2"
  Bus Creator1/1 -> Bus Creator2/2  "Status 1"
  Bus Creator2/1 -> IPT/1  "IPT"
  Bus Creator3/1 -> Bus Creator2/3  "ID"
  Bus Creator4/1 -> Bus Creator2/4  "DCDC_Status"
  Compare To Constant/1 -> motohawk_fault_def/1  "AgeCount"
  Read CAN Message/2 -> Bus Creator/1, motohawk_probe/1  "Torque Delivered"
  Read CAN Message/3 -> Bus Creator/2, motohawk_probe1/1  "DC Current"
  Read CAN Message/5 -> motohawk_probe3/1, Bus Creator/4, speed_calc/1(whl_rpm)  "Motor Speed"
  Read CAN Message/1 -> Compare To Constant/1  "AgeCount"
  Read CAN Message/4 -> Bus Creator/3, motohawk_probe2/1  "DC Voltage"
  Compare To Constant1/1 -> motohawk_fault_def1/1  "AgeCount"
  Read CAN Message1/1 -> Compare To Constant1/1  "AgeCount"
  Read CAN Message1/2 -> motohawk_probe4/1, Bus Creator1/1  "MCU Ready"
  Read CAN Message1/3 -> motohawk_probe5/1  "Derated Operation"
  Read CAN Message1/4 -> motohawk_probe6/1  "E-Drive System Error"
  Read CAN Message1/5 -> motohawk_probe7/1  "Emergency Shutdown"
  Read CAN Message1/6 -> motohawk_probe8/1  "Over Current IGBT Error"
  Read CAN Message1/7 -> motohawk_probe9/1  "Lube(Anal) Error"
  Read CAN Message1/8 -> motohawk_probe10/1  "Encoder Error"
  Read CAN Message1/9 -> motohawk_probe11/1  "OverVoltage Error"
  Read CAN Message1/10 -> motohawk_probe12/1  "UnderVoltage Error"
  Read CAN Message1/11 -> motohawk_probe13/1  "OverCurrent-AC Error"
  Read CAN Message1/12 -> motohawk_probe14/1  "Motor OverTemp"
  Read CAN Message1/13 -> motohawk_probe15/1  "Inverter OverTemp"
  Read CAN Message1/14 -> motohawk_probe16/1  "OverSpeed Error"
  Read CAN Message1/15 -> motohawk_probe66/1  "CAN Error"
  Read CAN Message1/16 -> motohawk_probe18/1  "Unreasonable Limits"
  Read CAN Message1/17 -> motohawk_probe19/1  "EPO Line Error"
  Read CAN Message1/18 -> motohawk_probe20/1  "Sensor Out Of Range"
  Read CAN Message1/19 -> motohawk_probe21/1  "Voltage Limitation active"
  Read CAN Message1/20 -> motohawk_probe22/1  "Current Limitiation active"
  Read CAN Message1/21 -> motohawk_probe23/1  "Pull Out Torque Protection active"
  Read CAN Message1/22 -> motohawk_probe24/1  "Peak Level Overflow"
  Read CAN Message1/23 -> motohawk_probe25/1  "Parity bit phase current"
  Read CAN Message1/24 -> motohawk_probe26/1  "Phase Current Peak-Value"
  Read CAN Message1/25 -> motohawk_probe27/1, Bus Creator1/2  "Max Torque available"
  Read CAN Message1/26 -> motohawk_probe28/1, Bus Creator1/3  "MCU Ready to Go"
  Read CAN Message1/27 -> motohawk_probe29/1  "MCU Hardware/Software Error"
  Read CAN Message1/28 -> motohawk_probe30/1  "MCU Speed Error Track Missing"
  Read CAN Message1/29 -> motohawk_probe31/1  "MCU Speed Error Speed Jump"
  Read CAN Message1/30 -> motohawk_probe32/1  "Error in Error Store"
  Read CAN Message1/31 -> motohawk_probe33/1  "Supply Line Low Error"
  Read CAN Message1/32 -> motohawk_probe34/1  "MCU On"
  Compare To Constant2/1 -> motohawk_fault_def2/1  "AgeCount"
  Read CAN Message2/1 -> Compare To Constant2/1  "AgeCount"
  Read CAN Message2/2 -> motohawk_probe35/1  "Sw_Ver"
  Read CAN Message2/3 -> motohawk_probe36/1  "IPT_Ser_Num"
  Read CAN Message2/4 -> motohawk_probe37/1, Bus Creator3/1, [Gear_Ratio]  "Gear_Ratio"
  Read CAN Message2/5 -> motohawk_probe38/1  "Oil_Pressure"
  Read CAN Message2/6 -> motohawk_probe39/1  "Motor_Temp"
  Read CAN Message2/7 -> motohawk_probe40/1  "MCU_Temp"
  Compare To Constant3/1 -> motohawk_fault_def3/1  "AgeCount"
  Read CAN Message3/1 -> Compare To Constant3/1  "AgeCount"
  Read CAN Message3/2 -> motohawk_probe41/1, Bus Creator4/1  "LV_Current"
  Read CAN Message3/3 -> motohawk_probe42/1, Bus Creator4/2  "LV_Voltage"
  Read CAN Message3/4 -> motohawk_probe43/1, Bus Creator4/3  "HV_DCDC_Current"
  Read CAN Message3/5 -> motohawk_probe44/1  "DCDC_GenError"
  Read CAN Message3/6 -> motohawk_probe45/1  "DCDC_HV_Over_I"
  Read CAN Message3/7 -> motohawk_probe46/1  "DCDC_HV_Over_V"
  Read CAN Message3/8 -> motohawk_probe47/1  "DCDC_LV_Over_I_Buck"
  Read CAN Message3/9 -> motohawk_probe48/1  "DCDC_LV_Under_V"
  Read CAN Message3/10 -> motohawk_probe49/1  "DCDC_LV_Over_V"
  Read CAN Message3/11 -> motohawk_probe50/1  "DCDC_LV_Over_I_Boost"
  Read CAN Message3/12 -> motohawk_probe51/1  "DCDC_Temp_Reduction"
  Read CAN Message3/13 -> motohawk_probe52/1  "DCDC_Buck"
  Read CAN Message3/14 -> motohawk_probe53/1  "DCDC_Boost"
  Read CAN Message3/15 -> motohawk_probe54/1  "DCDC_Reduce_Buck"
  Read CAN Message3/16 -> motohawk_probe55/1  "DCDC_Reduce_Boost"
  Read CAN Message3/17 -> motohawk_probe56/1  "DCDC_CAN_Err"
  Read CAN Message3/18 -> motohawk_probe57/1  "DCDC_Meas_Err"
  Read CAN Message3/19 -> motohawk_probe58/1  "DCDC_OverTemp"
  Read CAN Message3/20 -> motohawk_probe59/1  "DCDC_90I2t"
  Read CAN Message3/21 -> motohawk_probe60/1  "DCDC_Break"
  Read CAN Message3/22 -> motohawk_probe61/1  "DCDC_3x_En"
  Read CAN Message3/23 -> motohawk_probe62/1  "DCDC_>0C"
  Read CAN Message3/24 -> motohawk_probe63/1  "DCDC_HV_Under_V"
  Read CAN Message3/25 -> motohawk_probe64/1  "DCDC_HW_Err"
  Read CAN Message3/26 -> motohawk_probe65/1  "DCDC_Err_in_Store"
  speed_calc/1(Veh_mph) -> Bus Creator/5, motohawk_probe17/1  "veh_speed"
  [Gear_Ratio] -> speed_calc/2(gear_ratio)

== system cx06_MA/Inputs/JCI CAN Input ==
  Bus Creator3 : BusCreator
  Read CAN Message : MotoHawk_lib/CAN Blocks/Read CAN Message  nam=['CAN_' num2str(2)]  bus=-2  msg=CANRx_JCS_300  queue=1  slot=''  valid=off  stale=off  labelwires=on
  Read CAN Message1 : MotoHawk_lib/CAN Blocks/Read CAN Message  nam=['CAN_' num2str(2)]  bus=-2  msg=CANRx_JCS_310  queue=2  slot=''  valid=off  stale=off  labelwires=on
  SOC : Stateflow chart  TreatAsAtomicUnit=on
  Unit Delay : UnitDelay  SampleTime=-1
  motohawk_calibration : MotoHawk_lib/Calibration & Probing Blocks/motohawk_calibration  nam='cuurentPlusMinus'  val=3.25  storage=Calibration  show_more=on  name_source=Use Parameter  data_type=double  read_level=1  write_level=1  ovr_cals=on  view_as=Number  enum_struct={'Disabled', 'Enabled'}  vector_style=Wide Row  use_help_units=off  help=''  units=''  use_header_enum=off  row_header_enum={}  col_header_enum={}  use_min_max=off  min_val=-inf  max_val=inf  use_precision=off  precision=''  gain=1  offset=0  exp=1  use_mototune_group=off  mototune_group=motohawk_vardec_path(gcb)
  motohawk_calibration1 : MotoHawk_lib/Calibration & Probing Blocks/motohawk_calibration  nam='lowV'  val=195  storage=Calibration  show_more=on  name_source=Use Parameter  data_type=double  read_level=1  write_level=1  ovr_cals=on  view_as=Number  enum_struct={'Disabled', 'Enabled'}  vector_style=Wide Row  use_help_units=off  help=''  units=''  use_header_enum=off  row_header_enum={}  col_header_enum={}  use_min_max=off  min_val=-inf  max_val=inf  use_precision=off  precision=''  gain=1  offset=0  exp=1  use_mototune_group=off  mototune_group=motohawk_vardec_path(gcb)
  motohawk_calibration2 : MotoHawk_lib/Calibration & Probing Blocks/motohawk_calibration  nam='highV'  val=285  storage=Calibration  show_more=on  name_source=Use Parameter  data_type=double  read_level=1  write_level=1  ovr_cals=on  view_as=Number  enum_struct={'Disabled', 'Enabled'}  vector_style=Wide Row  use_help_units=off  help=''  units=''  use_header_enum=off  row_header_enum={}  col_header_enum={}  use_min_max=off  min_val=-inf  max_val=inf  use_precision=off  precision=''  gain=1  offset=0  exp=1  use_mototune_group=off  mototune_group=motohawk_vardec_path(gcb)
  motohawk_probe{,1..3} (4 alike) : MotoHawk_lib/Calibration & Probing Blocks/motohawk_probe  nam='Probe'  show_more=on  name_source=Use Input Wire Name  read_level=1  view_as=Number  enum_struct={'Disabled', 'Enabled'}  vector_style=Wide Row  use_help_units=off  help=''  units=''  use_header_enum=off  row_header_enum={}  col_header_enum={}  use_precision=off  precision=''  gain=1  offset=0  exp=1  use_mototune_group=off  mototune_group=motohawk_vardec_path(gcb)
  JCI : Outport  OutDataType=sfix(16)  OutScaling=2^0
  wires:
  Bus Creator3/1 -> JCI/1  "JCI"
  Read CAN Message/1 -> Bus Creator3/2, SOC/1(voltage), motohawk_probe/1  "Voltage"
  Read CAN Message/2 -> motohawk_probe1/1, Bus Creator3/3, SOC/5(currentBat)  "Current"
  Read CAN Message1/1 -> motohawk_probe2/1, Bus Creator3/4  "Batt_Temp"
  SOC/1(SOC) -> Unit Delay/1, Bus Creator3/1, motohawk_probe3/1  "SOC"
  motohawk_calibration/1 -> SOC/2(currentPlusMinus)
  motohawk_calibration2/1 -> SOC/4(highV)
  motohawk_calibration1/1 -> SOC/3(lowV)
  Unit Delay/1 -> SOC/6(SOCLast)
